simulink model "FilterBlock"  (R2020b)
settings: Solver=FixedStepAuto  StartTime=0.0  StopTime=10  FixedStep=0.2  RelTol=1e-3
settings Model: Creator=BIDITA PAUL  LastModifiedBy=BIDITA PAUL
settings DataIOCC: SaveOutput=off  SaveTime=off

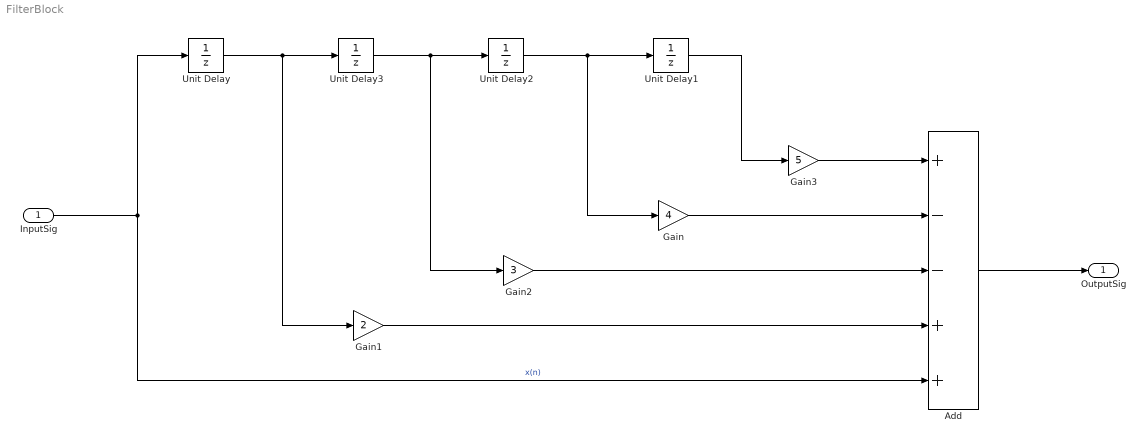
== system FilterBlock ==
  InputSig : Inport  OutDataTypeStr=double  PortDimensions=1
  Add : Sum  Inputs=+--++
  Gain : Gain  Gain=4
  Gain1 : Gain  Gain=2
  Gain2 : Gain  Gain=3
  Gain3 : Gain  Gain=5
  Unit Delay{,1..3} (4 alike) : UnitDelay  SampleTime=-1  HasFrameUpgradeWarning=on
  OutputSig : Outport  OutDataTypeStr=double  PortDimensions=1  SampleTime=[0.20000000000000001,0]
  wires:
  Unit Delay/1 -> Unit Delay3/1, Gain1/1
  Gain2/1 -> Add/3
  Unit Delay1/1 -> Gain3/1
  Unit Delay2/1 -> Unit Delay1/1, Gain/1
  Gain/1 -> Add/2
  Unit Delay3/1 -> Unit Delay2/1, Gain2/1
  Gain3/1 -> Add/1
  Gain1/1 -> Add/4
  InputSig/1 -> Add/5, Unit Delay/1  "x(n)"
  Add/1 -> OutputSig/1
